simulink library "tenneco_lib"  (R2016b)
settings: Solver=ode45  StartTime=0.0  StopTime=10.0  RelTol=1e-3
undefined symbols (not defined in the file): Com_cntAMBInitTO_c, Com_cntAMBStopTO_c, Com_cntEC1InitTO_c, Com_cntEC1StopTO_c, Com_swAMBRx_c, Com_swEC1Rx_c, Com_swUseSPN108_c, Com_swUseSPN543_c, const, Env_pAmbPDflt_c, Env_pAmbPKOff_c, Env_pAmbPOvrd_c, Env_swAmbPOvrd_c, MSG_INIT_TIMEOUT, MSG_NOT_RECEIVED, MSG_RECEIVED_NOW, MSG_STOP_TIMEOUT
libraries: simulink x19, tenneco_lib x2
(part 3 of 5)

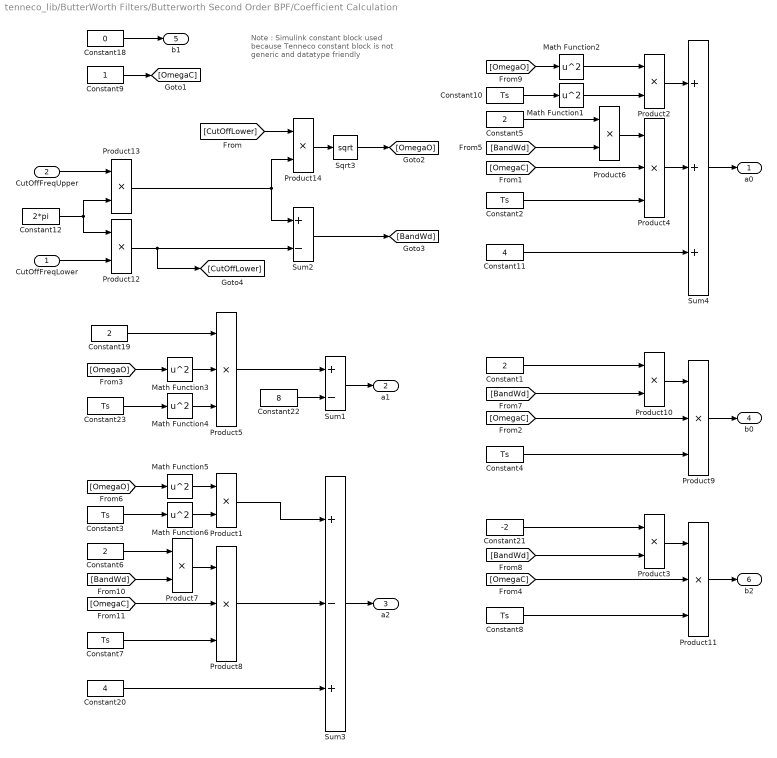
== system tenneco_lib/ButterWorth Filters/Butterworth Second Order BPF/Coefficient Calculation ==
  note: Note : Simulink constant block used because Tenneco constant block is not generic and datatype friendly
  CutOffFreqLower : Inport  mask(Standard Inport){Port=1}
      mask prompts: Port "Simulink:blkprm_prompts:InOutportPortNum"
      mask help: Provide an input port for subsystems.
      mask TypeOptions Port: Port
  CutOffFreqUpper : Inport  Port=2  mask(Standard Inport){Port=2}
      mask prompts: Port "Simulink:blkprm_prompts:InOutportPortNum"
      mask help: Provide an input port for subsystems.
      mask TypeOptions Port: Port
  Constant{1,5..6,19} (4 alike) : Constant  Value=2  OutDataTypeStr=Inherit: Inherit via back propagation
  Constant{2..4,7..8,10,23} (7 alike) : Constant  Value=Ts  OutDataTypeStr=Inherit: Inherit via back propagation
  Constant11 : Constant  Value=4  OutDataTypeStr=Inherit: Inherit via back propagation
  Constant12 : Constant  Value=2*pi  OutDataTypeStr=Inherit: Inherit via back propagation
  Constant18 : Constant  Value=0  OutDataTypeStr=Inherit: Inherit via back propagation
  Constant20 : Constant  Value=4  OutDataTypeStr=Inherit: Inherit via back propagation
  Constant21 : Constant  Value=-2  OutDataTypeStr=Inherit: Inherit via back propagation
  Constant22 : Constant  Value=8  OutDataTypeStr=Inherit: Inherit via back propagation
  Constant9 : Constant  OutDataTypeStr=Inherit: Inherit via back propagation
  Math Function1 : Math  Operator=square  SaturateOnIntegerOverflow=on  mask(Math){Operator=square}
      mask prompts: Operator "SimulinkBlocks:dialog:BmathfcnOperator"
      mask help: Mathematical functions including logarithmic, exponential, power, and modulus functions. When the function has more than one argument, the first argument corresponds to the top (or left) input port.
      mask TypeOptions Operator: Operator
  Math Function2 : Math  Operator=square  SaturateOnIntegerOverflow=on  mask(Math){Operator=square}
      mask prompts: Operator "SimulinkBlocks:dialog:BmathfcnOperator"
      mask help: Mathematical functions including logarithmic, exponential, power, and modulus functions. When the function has more than one argument, the first argument corresponds to the top (or left) input port.
      mask TypeOptions Operator: Operator
  Math Function3 : Math  Operator=square  SaturateOnIntegerOverflow=on  mask(Math){Operator=square}
      mask prompts: Operator "SimulinkBlocks:dialog:BmathfcnOperator"
      mask help: Mathematical functions including logarithmic, exponential, power, and modulus functions. When the function has more than one argument, the first argument corresponds to the top (or left) input port.
      mask TypeOptions Operator: Operator
  Math Function4 : Math  Operator=square  SaturateOnIntegerOverflow=on  mask(Math){Operator=square}
      mask prompts: Operator "SimulinkBlocks:dialog:BmathfcnOperator"
      mask help: Mathematical functions including logarithmic, exponential, power, and modulus functions. When the function has more than one argument, the first argument corresponds to the top (or left) input port.
      mask TypeOptions Operator: Operator
  Math Function5 : Math  Operator=square  SaturateOnIntegerOverflow=on  mask(Math){Operator=square}
      mask prompts: Operator "SimulinkBlocks:dialog:BmathfcnOperator"
      mask help: Mathematical functions including logarithmic, exponential, power, and modulus functions. When the function has more than one argument, the first argument corresponds to the top (or left) input port.
      mask TypeOptions Operator: Operator
  Math Function6 : Math  Operator=square  SaturateOnIntegerOverflow=on  mask(Math){Operator=square}
      mask prompts: Operator "SimulinkBlocks:dialog:BmathfcnOperator"
      mask help: Mathematical functions including logarithmic, exponential, power, and modulus functions. When the function has more than one argument, the first argument corresponds to the top (or left) input port.
      mask TypeOptions Operator: Operator
  Product1 : Product  Inputs=**  InputSameDT=on  mask(Product){Inputs=**}
      mask prompts: Inputs "List of signs:"
      mask help:
      | Multiply or divide inputs.  Specify one of the following:
      |  a) * or / for each input port. For example, **/* performs the operation 'u1*u2/u3*u4'.
      |  b) scalar specifies the number of input ports to be multiplied.
      mask TypeOptions Inputs: Inputs
  Product10 : Product  Inputs=**  InputSameDT=on  mask(Product){Inputs=**}
      mask prompts: Inputs "List of signs:"
      mask help:
      | Multiply or divide inputs.  Specify one of the following:
      |  a) * or / for each input port. For example, **/* performs the operation 'u1*u2/u3*u4'.
      |  b) scalar specifies the number of input ports to be multiplied.
      mask TypeOptions Inputs: Inputs
  Product11 : Product  Inputs=***  InputSameDT=on  mask(Product){Inputs=***}
      mask prompts: Inputs "List of signs:"
      mask help:
      | Multiply or divide inputs.  Specify one of the following:
      |  a) * or / for each input port. For example, **/* performs the operation 'u1*u2/u3*u4'.
      |  b) scalar specifies the number of input ports to be multiplied.
      mask TypeOptions Inputs: Inputs
  Product12 : Product  Inputs=**  InputSameDT=on  mask(Product){Inputs=**}
      mask prompts: Inputs "List of signs:"
      mask help:
      | Multiply or divide inputs.  Specify one of the following:
      |  a) * or / for each input port. For example, **/* performs the operation 'u1*u2/u3*u4'.
      |  b) scalar specifies the number of input ports to be multiplied.
      mask TypeOptions Inputs: Inputs
  Product13 : Product  Inputs=**  InputSameDT=on  mask(Product){Inputs=**}
      mask prompts: Inputs "List of signs:"
      mask help:
      | Multiply or divide inputs.  Specify one of the following:
      |  a) * or / for each input port. For example, **/* performs the operation 'u1*u2/u3*u4'.
      |  b) scalar specifies the number of input ports to be multiplied.
      mask TypeOptions Inputs: Inputs
  Product14 : Product  Inputs=**  InputSameDT=on  mask(Product){Inputs=**}
      mask prompts: Inputs "List of signs:"
      mask help:
      | Multiply or divide inputs.  Specify one of the following:
      |  a) * or / for each input port. For example, **/* performs the operation 'u1*u2/u3*u4'.
      |  b) scalar specifies the number of input ports to be multiplied.
      mask TypeOptions Inputs: Inputs
  Product2 : Product  Inputs=**  InputSameDT=on  mask(Product){Inputs=**}
      mask prompts: Inputs "List of signs:"
      mask help:
      | Multiply or divide inputs.  Specify one of the following:
      |  a) * or / for each input port. For example, **/* performs the operation 'u1*u2/u3*u4'.
      |  b) scalar specifies the number of input ports to be multiplied.
      mask TypeOptions Inputs: Inputs
  Product3 : Product  Inputs=**  InputSameDT=on  mask(Product){Inputs=**}
      mask prompts: Inputs "List of signs:"
      mask help:
      | Multiply or divide inputs.  Specify one of the following:
      |  a) * or / for each input port. For example, **/* performs the operation 'u1*u2/u3*u4'.
      |  b) scalar specifies the number of input ports to be multiplied.
      mask TypeOptions Inputs: Inputs
  Product4 : Product  Inputs=***  InputSameDT=on  mask(Product){Inputs=***}
      mask prompts: Inputs "List of signs:"
      mask help:
      | Multiply or divide inputs.  Specify one of the following:
      |  a) * or / for each input port. For example, **/* performs the operation 'u1*u2/u3*u4'.
      |  b) scalar specifies the number of input ports to be multiplied.
      mask TypeOptions Inputs: Inputs
  Product5 : Product  Inputs=***  InputSameDT=on  mask(Product){Inputs=***}
      mask prompts: Inputs "List of signs:"
      mask help:
      | Multiply or divide inputs.  Specify one of the following:
      |  a) * or / for each input port. For example, **/* performs the operation 'u1*u2/u3*u4'.
      |  b) scalar specifies the number of input ports to be multiplied.
      mask TypeOptions Inputs: Inputs
  Product6 : Product  Inputs=**  InputSameDT=on  mask(Product){Inputs=**}
      mask prompts: Inputs "List of signs:"
      mask help:
      | Multiply or divide inputs.  Specify one of the following:
      |  a) * or / for each input port. For example, **/* performs the operation 'u1*u2/u3*u4'.
      |  b) scalar specifies the number of input ports to be multiplied.
      mask TypeOptions Inputs: Inputs
  Product7 : Product  Inputs=**  InputSameDT=on  mask(Product){Inputs=**}
      mask prompts: Inputs "List of signs:"
      mask help:
      | Multiply or divide inputs.  Specify one of the following:
      |  a) * or / for each input port. For example, **/* performs the operation 'u1*u2/u3*u4'.
      |  b) scalar specifies the number of input ports to be multiplied.
      mask TypeOptions Inputs: Inputs
  Product8 : Product  Inputs=***  InputSameDT=on  mask(Product){Inputs=***}
      mask prompts: Inputs "List of signs:"
      mask help:
      | Multiply or divide inputs.  Specify one of the following:
      |  a) * or / for each input port. For example, **/* performs the operation 'u1*u2/u3*u4'.
      |  b) scalar specifies the number of input ports to be multiplied.
      mask TypeOptions Inputs: Inputs
  Product9 : Product  Inputs=***  InputSameDT=on  mask(Product){Inputs=***}
      mask prompts: Inputs "List of signs:"
      mask help:
      | Multiply or divide inputs.  Specify one of the following:
      |  a) * or / for each input port. For example, **/* performs the operation 'u1*u2/u3*u4'.
      |  b) scalar specifies the number of input ports to be multiplied.
      mask TypeOptions Inputs: Inputs
  Sqrt3 : Sqrt  SaturateOnIntegerOverflow=on  mask(Sqrt){Operator=sqrt}
      mask prompts: Operator "SimulinkBlocks:SqrtFcn:BmathfcnOperator"
      mask help: Square root functions including square root, signed square root, and reciprocal square root functions.
      mask TypeOptions Operator: Operator
  Sum1 : Sum  Inputs=+-  InputSameDT=on  mask(Sum){Inputs=+-}
      mask prompts: Inputs "Simulink:blkprm_prompts:SumListofSigns"
      mask help:
      | Add or subtract inputs.  Specify one of the following:
      | a) character vector containing + or - for each input port, | for spacer between ports (e.g. ++|-|++)
      | b) scalar, >= 1, specifies the number of input ports to be summed.
      | When there is only one input port, add or subtract elements over all dimensions or one specified dimension
      mask TypeOptions Inputs: Inputs
  Sum2 : Sum  Inputs=+-  InputSameDT=on  mask(Sum){Inputs=+-}
      mask prompts: Inputs "Simulink:blkprm_prompts:SumListofSigns"
      mask help:
      | Add or subtract inputs.  Specify one of the following:
      | a) character vector containing + or - for each input port, | for spacer between ports (e.g. ++|-|++)
      | b) scalar, >= 1, specifies the number of input ports to be summed.
      | When there is only one input port, add or subtract elements over all dimensions or one specified dimension
      mask TypeOptions Inputs: Inputs
  Sum3 : Sum  Inputs=+-+  InputSameDT=on  mask(Sum){Inputs=+-+}
      mask prompts: Inputs "Simulink:blkprm_prompts:SumListofSigns"
      mask help:
      | Add or subtract inputs.  Specify one of the following:
      | a) character vector containing + or - for each input port, | for spacer between ports (e.g. ++|-|++)
      | b) scalar, >= 1, specifies the number of input ports to be summed.
      | When there is only one input port, add or subtract elements over all dimensions or one specified dimension
      mask TypeOptions Inputs: Inputs
  Sum4 : Sum  Inputs=+++  InputSameDT=on  mask(Sum){Inputs=+++}
      mask prompts: Inputs "Simulink:blkprm_prompts:SumListofSigns"
      mask help:
      | Add or subtract inputs.  Specify one of the following:
      | a) character vector containing + or - for each input port, | for spacer between ports (e.g. ++|-|++)
      | b) scalar, >= 1, specifies the number of input ports to be summed.
      | When there is only one input port, add or subtract elements over all dimensions or one specified dimension
      mask TypeOptions Inputs: Inputs
  a0 : Outport  mask(Standard Outport){Port=1}
      mask prompts: Port "Simulink:blkprm_prompts:InOutportPortNum"
      mask help: Provide an output port for subsystems.
      mask TypeOptions Port: Port
  a1 : Outport  Port=2  mask(Standard Outport){Port=2}
      mask prompts: Port "Simulink:blkprm_prompts:InOutportPortNum"
      mask help: Provide an output port for subsystems.
      mask TypeOptions Port: Port
  a2 : Outport  Port=3  mask(Standard Outport){Port=3}
      mask prompts: Port "Simulink:blkprm_prompts:InOutportPortNum"
      mask help: Provide an output port for subsystems.
      mask TypeOptions Port: Port
  b0 : Outport  Port=4  mask(Standard Outport){Port=4}
      mask prompts: Port "Simulink:blkprm_prompts:InOutportPortNum"
      mask help: Provide an output port for subsystems.
      mask TypeOptions Port: Port
  b1 : Outport  Port=5  mask(Standard Outport){Port=5}
      mask prompts: Port "Simulink:blkprm_prompts:InOutportPortNum"
      mask help: Provide an output port for subsystems.
      mask TypeOptions Port: Port
  b2 : Outport  Port=6  mask(Standard Outport){Port=6}
      mask prompts: Port "Simulink:blkprm_prompts:InOutportPortNum"
      mask help: Provide an output port for subsystems.
      mask TypeOptions Port: Port
  wires:
  Constant18/1 -> b1/1
  Sum1/1 -> a1/1
  Constant9/1 -> [OmegaC]
  [OmegaO] -> Math Function2/1
  Product2/1 -> Sum4/1
  Math Function2/1 -> Product2/1
  Math Function1/1 -> Product2/2
  Constant10/1 -> Math Function1/1
  Constant11/1 -> Sum4/3
  Product4/1 -> Sum4/2
  [OmegaC] -> Product4/2
  Constant2/1 -> Product4/3
  Product6/1 -> Product4/1
  Constant5/1 -> Product6/1
  [BandWd] -> Product6/2
  Sum4/1 -> a0/1
  Constant22/1 -> Sum1/2
  [OmegaO] -> Math Function3/1
  Product5/1 -> Sum1/1
  Constant23/1 -> Math Function4/1
  Math Function3/1 -> Product5/2
  Math Function4/1 -> Product5/3
  Constant19/1 -> Product5/1
  [OmegaO] -> Math Function5/1
  Product1/1 -> Sum3/1
  Math Function5/1 -> Product1/1
  Math Function6/1 -> Product1/2
  Constant3/1 -> Math Function6/1
  Constant20/1 -> Sum3/3
  Product8/1 -> Sum3/2
  [OmegaC] -> Product8/2
  Constant7/1 -> Product8/3
  Product7/1 -> Product8/1
  Constant6/1 -> Product7/1
  [BandWd] -> Product7/2
  Sum3/1 -> a2/1
  Product9/1 -> b0/1
  [OmegaC] -> Product9/2
  Constant4/1 -> Product9/3
  Product10/1 -> Product9/1
  [BandWd] -> Product10/2
  Constant1/1 -> Product10/1
  Product11/1 -> b2/1
  [OmegaC] -> Product11/2
  Constant8/1 -> Product11/3
  Product3/1 -> Product11/1
  [BandWd] -> Product3/2
  Constant21/1 -> Product3/1
  Sqrt3/1 -> [OmegaO]
  Product14/1 -> Sqrt3/1
  [CutOffLower] -> Product14/1
  Sum2/1 -> [BandWd]
  Product12/1 -> Sum2/2, [CutOffLower]
  Product13/1 -> Sum2/1, Product14/2
  CutOffFreqLower/1 -> Product12/2
  CutOffFreqUpper/1 -> Product13/1
  Constant12/1 -> Product13/2, Product12/1

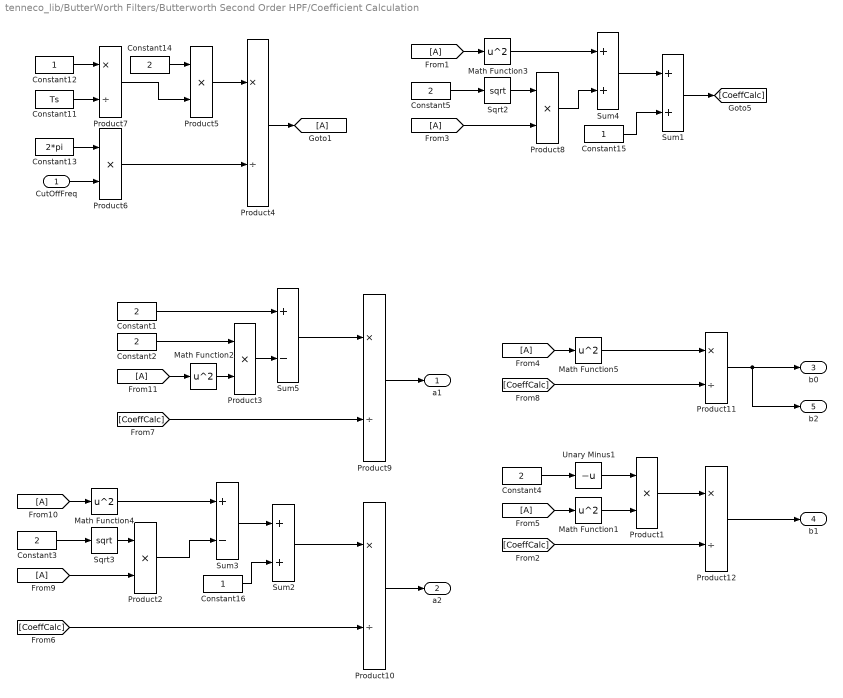
== system tenneco_lib/ButterWorth Filters/Butterworth Second Order HPF/Coefficient Calculation ==
  CutOffFreq : Inport  mask(Standard Inport){Port=1}
      mask prompts: Port "Simulink:blkprm_prompts:InOutportPortNum"
      mask help: Provide an input port for subsystems.
      mask TypeOptions Port: Port
  Constant{1..5,14} (6 alike) : Constant  Value=2  OutDataTypeStr=Inherit: Inherit via back propagation
  Constant11 : Constant  Value=Ts  OutDataTypeStr=Inherit: Inherit via back propagation
  Constant12 : Constant  OutDataTypeStr=Inherit: Inherit via back propagation
  Constant13 : Constant  Value=2*pi  OutDataTypeStr=Inherit: Inherit via back propagation
  Constant15 : Constant  OutDataTypeStr=Inherit: Inherit via back propagation
  Constant16 : Constant  OutDataTypeStr=Inherit: Inherit via back propagation
  Math Function1 : Math  Operator=square  SaturateOnIntegerOverflow=on  mask(Math){Operator=square}
      mask prompts: Operator "SimulinkBlocks:dialog:BmathfcnOperator"
      mask help: Mathematical functions including logarithmic, exponential, power, and modulus functions. When the function has more than one argument, the first argument corresponds to the top (or left) input port.
      mask TypeOptions Operator: Operator
  Math Function2 : Math  Operator=square  SaturateOnIntegerOverflow=on  mask(Math){Operator=square}
      mask prompts: Operator "SimulinkBlocks:dialog:BmathfcnOperator"
      mask help: Mathematical functions including logarithmic, exponential, power, and modulus functions. When the function has more than one argument, the first argument corresponds to the top (or left) input port.
      mask TypeOptions Operator: Operator
  Math Function3 : Math  Operator=square  SaturateOnIntegerOverflow=on  mask(Math){Operator=square}
      mask prompts: Operator "SimulinkBlocks:dialog:BmathfcnOperator"
      mask help: Mathematical functions including logarithmic, exponential, power, and modulus functions. When the function has more than one argument, the first argument corresponds to the top (or left) input port.
      mask TypeOptions Operator: Operator
  Math Function4 : Math  Operator=square  SaturateOnIntegerOverflow=on  mask(Math){Operator=square}
      mask prompts: Operator "SimulinkBlocks:dialog:BmathfcnOperator"
      mask help: Mathematical functions including logarithmic, exponential, power, and modulus functions. When the function has more than one argument, the first argument corresponds to the top (or left) input port.
      mask TypeOptions Operator: Operator
  Math Function5 : Math  Operator=square  SaturateOnIntegerOverflow=on  mask(Math){Operator=square}
      mask prompts: Operator "SimulinkBlocks:dialog:BmathfcnOperator"
      mask help: Mathematical functions including logarithmic, exponential, power, and modulus functions. When the function has more than one argument, the first argument corresponds to the top (or left) input port.
      mask TypeOptions Operator: Operator
  Product1 : Product  Inputs=**  InputSameDT=on  mask(Product){Inputs=**}
      mask prompts: Inputs "List of signs:"
      mask help:
      | Multiply or divide inputs.  Specify one of the following:
      |  a) * or / for each input port. For example, **/* performs the operation 'u1*u2/u3*u4'.
      |  b) scalar specifies the number of input ports to be multiplied.
      mask TypeOptions Inputs: Inputs
  Product10 : Product  Inputs=*/  InputSameDT=on  mask(Product){Inputs=*/}
      mask prompts: Inputs "List of signs:"
      mask help:
      | Multiply or divide inputs.  Specify one of the following:
      |  a) * or / for each input port. For example, **/* performs the operation 'u1*u2/u3*u4'.
      |  b) scalar specifies the number of input ports to be multiplied.
      mask TypeOptions Inputs: Inputs
  Product11 : Product  Inputs=*/  InputSameDT=on  mask(Product){Inputs=*/}
      mask prompts: Inputs "List of signs:"
      mask help:
      | Multiply or divide inputs.  Specify one of the following:
      |  a) * or / for each input port. For example, **/* performs the operation 'u1*u2/u3*u4'.
      |  b) scalar specifies the number of input ports to be multiplied.
      mask TypeOptions Inputs: Inputs
  Product12 : Product  Inputs=*/  InputSameDT=on  mask(Product){Inputs=*/}
      mask prompts: Inputs "List of signs:"
      mask help:
      | Multiply or divide inputs.  Specify one of the following:
      |  a) * or / for each input port. For example, **/* performs the operation 'u1*u2/u3*u4'.
      |  b) scalar specifies the number of input ports to be multiplied.
      mask TypeOptions Inputs: Inputs
  Product2 : Product  Inputs=**  InputSameDT=on  mask(Product){Inputs=**}
      mask prompts: Inputs "List of signs:"
      mask help:
      | Multiply or divide inputs.  Specify one of the following:
      |  a) * or / for each input port. For example, **/* performs the operation 'u1*u2/u3*u4'.
      |  b) scalar specifies the number of input ports to be multiplied.
      mask TypeOptions Inputs: Inputs
  Product3 : Product  Inputs=**  InputSameDT=on  mask(Product){Inputs=**}
      mask prompts: Inputs "List of signs:"
      mask help:
      | Multiply or divide inputs.  Specify one of the following:
      |  a) * or / for each input port. For example, **/* performs the operation 'u1*u2/u3*u4'.
      |  b) scalar specifies the number of input ports to be multiplied.
      mask TypeOptions Inputs: Inputs
  Product4 : Product  Inputs=*/  InputSameDT=on  mask(Product){Inputs=*/}
      mask prompts: Inputs "List of signs:"
      mask help:
      | Multiply or divide inputs.  Specify one of the following:
      |  a) * or / for each input port. For example, **/* performs the operation 'u1*u2/u3*u4'.
      |  b) scalar specifies the number of input ports to be multiplied.
      mask TypeOptions Inputs: Inputs
  Product5 : Product  Inputs=**  InputSameDT=on  mask(Product){Inputs=**}
      mask prompts: Inputs "List of signs:"
      mask help:
      | Multiply or divide inputs.  Specify one of the following:
      |  a) * or / for each input port. For example, **/* performs the operation 'u1*u2/u3*u4'.
      |  b) scalar specifies the number of input ports to be multiplied.
      mask TypeOptions Inputs: Inputs
  Product6 : Product  Inputs=**  InputSameDT=on  mask(Product){Inputs=**}
      mask prompts: Inputs "List of signs:"
      mask help:
      | Multiply or divide inputs.  Specify one of the following:
      |  a) * or / for each input port. For example, **/* performs the operation 'u1*u2/u3*u4'.
      |  b) scalar specifies the number of input ports to be multiplied.
      mask TypeOptions Inputs: Inputs
  Product7 : Product  Inputs=*/  InputSameDT=on  mask(Product){Inputs=*/}
      mask prompts: Inputs "List of signs:"
      mask help:
      | Multiply or divide inputs.  Specify one of the following:
      |  a) * or / for each input port. For example, **/* performs the operation 'u1*u2/u3*u4'.
      |  b) scalar specifies the number of input ports to be multiplied.
      mask TypeOptions Inputs: Inputs
  Product8 : Product  Inputs=**  InputSameDT=on  mask(Product){Inputs=**}
      mask prompts: Inputs "List of signs:"
      mask help:
      | Multiply or divide inputs.  Specify one of the following:
      |  a) * or / for each input port. For example, **/* performs the operation 'u1*u2/u3*u4'.
      |  b) scalar specifies the number of input ports to be multiplied.
      mask TypeOptions Inputs: Inputs
  Product9 : Product  Inputs=*/  InputSameDT=on  mask(Product){Inputs=*/}
      mask prompts: Inputs "List of signs:"
      mask help:
      | Multiply or divide inputs.  Specify one of the following:
      |  a) * or / for each input port. For example, **/* performs the operation 'u1*u2/u3*u4'.
      |  b) scalar specifies the number of input ports to be multiplied.
      mask TypeOptions Inputs: Inputs
  Sqrt2 : Sqrt  SaturateOnIntegerOverflow=on  mask(Sqrt){Operator=sqrt}
      mask prompts: Operator "SimulinkBlocks:SqrtFcn:BmathfcnOperator"
      mask help: Square root functions including square root, signed square root, and reciprocal square root functions.
      mask TypeOptions Operator: Operator
  Sqrt3 : Sqrt  SaturateOnIntegerOverflow=on  mask(Sqrt){Operator=sqrt}
      mask prompts: Operator "SimulinkBlocks:SqrtFcn:BmathfcnOperator"
      mask help: Square root functions including square root, signed square root, and reciprocal square root functions.
      mask TypeOptions Operator: Operator
  Sum1 : Sum  InputSameDT=on  mask(Sum){Inputs=++}
      mask prompts: Inputs "Simulink:blkprm_prompts:SumListofSigns"
      mask help:
      | Add or subtract inputs.  Specify one of the following:
      | a) character vector containing + or - for each input port, | for spacer between ports (e.g. ++|-|++)
      | b) scalar, >= 1, specifies the number of input ports to be summed.
      | When there is only one input port, add or subtract elements over all dimensions or one specified dimension
      mask TypeOptions Inputs: Inputs
  Sum2 : Sum  InputSameDT=on  mask(Sum){Inputs=++}
      mask prompts: Inputs "Simulink:blkprm_prompts:SumListofSigns"
      mask help:
      | Add or subtract inputs.  Specify one of the following:
      | a) character vector containing + or - for each input port, | for spacer between ports (e.g. ++|-|++)
      | b) scalar, >= 1, specifies the number of input ports to be summed.
      | When there is only one input port, add or subtract elements over all dimensions or one specified dimension
      mask TypeOptions Inputs: Inputs
  Sum3 : Sum  Inputs=+-  InputSameDT=on  mask(Sum){Inputs=+-}
      mask prompts: Inputs "Simulink:blkprm_prompts:SumListofSigns"
      mask help:
      | Add or subtract inputs.  Specify one of the following:
      | a) character vector containing + or - for each input port, | for spacer between ports (e.g. ++|-|++)
      | b) scalar, >= 1, specifies the number of input ports to be summed.
      | When there is only one input port, add or subtract elements over all dimensions or one specified dimension
      mask TypeOptions Inputs: Inputs
  Sum4 : Sum  InputSameDT=on  mask(Sum){Inputs=++}
      mask prompts: Inputs "Simulink:blkprm_prompts:SumListofSigns"
      mask help:
      | Add or subtract inputs.  Specify one of the following:
      | a) character vector containing + or - for each input port, | for spacer between ports (e.g. ++|-|++)
      | b) scalar, >= 1, specifies the number of input ports to be summed.
      | When there is only one input port, add or subtract elements over all dimensions or one specified dimension
      mask TypeOptions Inputs: Inputs
  Sum5 : Sum  Inputs=+-  InputSameDT=on  mask(Sum){Inputs=+-}
      mask prompts: Inputs "Simulink:blkprm_prompts:SumListofSigns"
      mask help:
      | Add or subtract inputs.  Specify one of the following:
      | a) character vector containing + or - for each input port, | for spacer between ports (e.g. ++|-|++)
      | b) scalar, >= 1, specifies the number of input ports to be summed.
      | When there is only one input port, add or subtract elements over all dimensions or one specified dimension
      mask TypeOptions Inputs: Inputs
  Unary Minus1 : UnaryMinus
  a1 : Outport  mask(Standard Outport){Port=1}
      mask prompts: Port "Simulink:blkprm_prompts:InOutportPortNum"
      mask help: Provide an output port for subsystems.
      mask TypeOptions Port: Port
  a2 : Outport  Port=2  mask(Standard Outport){Port=2}
      mask prompts: Port "Simulink:blkprm_prompts:InOutportPortNum"
      mask help: Provide an output port for subsystems.
      mask TypeOptions Port: Port
  b0 : Outport  Port=3  mask(Standard Outport){Port=3}
      mask prompts: Port "Simulink:blkprm_prompts:InOutportPortNum"
      mask help: Provide an output port for subsystems.
      mask TypeOptions Port: Port
  b1 : Outport  Port=4  mask(Standard Outport){Port=4}
      mask prompts: Port "Simulink:blkprm_prompts:InOutportPortNum"
      mask help: Provide an output port for subsystems.
      mask TypeOptions Port: Port
  b2 : Outport  Port=5  mask(Standard Outport){Port=5}
      mask prompts: Port "Simulink:blkprm_prompts:InOutportPortNum"
      mask help: Provide an output port for subsystems.
      mask TypeOptions Port: Port
  wires:
  Constant14/1 -> Product5/1
  Product7/1 -> Product5/2
  Product5/1 -> Product4/1
  Product4/1 -> [A]
  Product6/1 -> Product4/2
  Constant13/1 -> Product6/1
  Constant12/1 -> Product7/1
  CutOffFreq/1 -> Product6/2
  Constant11/1 -> Product7/2
  Unary Minus1/1 -> Product1/1
  Constant4/1 -> Unary Minus1/1
  Math Function1/1 -> Product1/2
  [A] -> Math Function1/1
  [A] -> Math Function5/1
  Product1/1 -> Product12/1
  [CoeffCalc] -> Product12/2
  Product12/1 -> b1/1
  [CoeffCalc] -> Product11/2
  [CoeffCalc] -> Product10/2
  [CoeffCalc] -> Product9/2
  Sum1/1 -> [CoeffCalc]
  Product10/1 -> a2/1
  Sum2/1 -> Product10/1
  Constant16/1 -> Sum2/2
  Sum3/1 -> Sum2/1
  Math Function4/1 -> Sum3/1
  Product2/1 -> Sum3/2
  [A] -> Product2/2
  Sqrt3/1 -> Product2/1
  Constant3/1 -> Sqrt3/1
  [A] -> Math Function4/1
  Product9/1 -> a1/1
  Constant15/1 -> Sum1/2
  Sum4/1 -> Sum1/1
  Math Function3/1 -> Sum4/1
  Product8/1 -> Sum4/2
  [A] -> Product8/2
  Sqrt2/1 -> Product8/1
  Constant5/1 -> Sqrt2/1
  [A] -> Math Function3/1
  Sum5/1 -> Product9/1
  Product3/1 -> Sum5/2
  Constant2/1 -> Product3/1
  Math Function2/1 -> Product3/2
  [A] -> Math Function2/1
  Constant1/1 -> Sum5/1
  Math Function5/1 -> Product11/1
  Product11/1 -> b2/1, b0/1

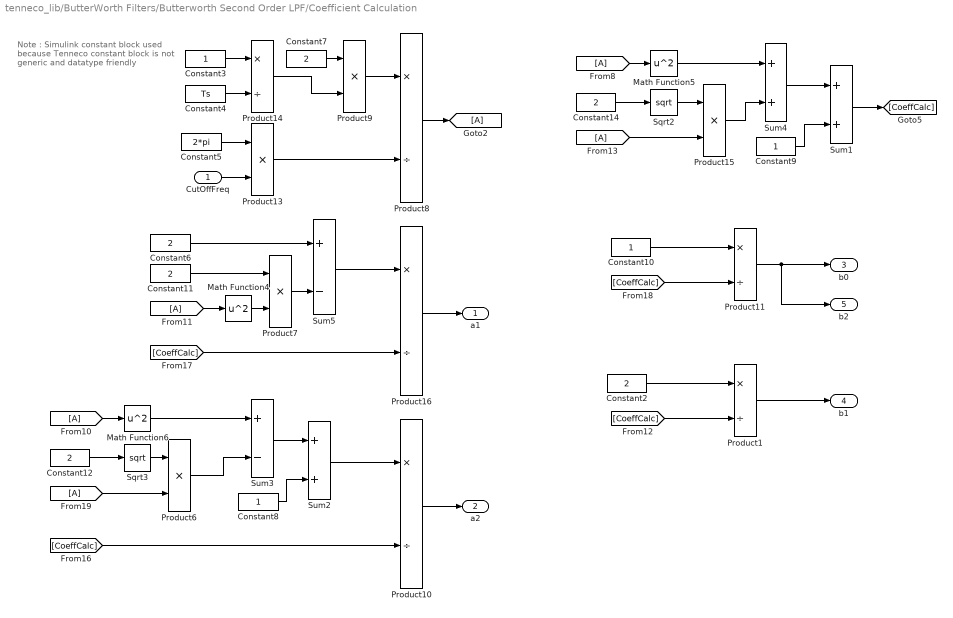
== system tenneco_lib/ButterWorth Filters/Butterworth Second Order LPF/Coefficient Calculation ==
  note: Note : Simulink constant block used because Tenneco constant block is not generic and datatype friendly
  CutOffFreq : Inport  mask(Standard Inport){Port=1}
      mask prompts: Port "Simulink:blkprm_prompts:InOutportPortNum"
      mask help: Provide an input port for subsystems.
      mask TypeOptions Port: Port
  Constant{3,8..10} (4 alike) : Constant  OutDataTypeStr=Inherit: Inherit via back propagation
  Constant{2,6..7,11..12,14} (6 alike) : Constant  Value=2  OutDataTypeStr=Inherit: Inherit via back propagation
  Constant4 : Constant  Value=Ts  OutDataTypeStr=Inherit: Inherit via back propagation
  Constant5 : Constant  Value=2*pi  OutDataTypeStr=Inherit: Inherit via back propagation
  Math Function4 : Math  Operator=square  SaturateOnIntegerOverflow=on  mask(Math){Operator=square}
      mask prompts: Operator "SimulinkBlocks:dialog:BmathfcnOperator"
      mask help: Mathematical functions including logarithmic, exponential, power, and modulus functions. When the function has more than one argument, the first argument corresponds to the top (or left) input port.
      mask TypeOptions Operator: Operator
  Math Function5 : Math  Operator=square  SaturateOnIntegerOverflow=on  mask(Math){Operator=square}
      mask prompts: Operator "SimulinkBlocks:dialog:BmathfcnOperator"
      mask help: Mathematical functions including logarithmic, exponential, power, and modulus functions. When the function has more than one argument, the first argument corresponds to the top (or left) input port.
      mask TypeOptions Operator: Operator
  Math Function6 : Math  Operator=square  SaturateOnIntegerOverflow=on  mask(Math){Operator=square}
      mask prompts: Operator "SimulinkBlocks:dialog:BmathfcnOperator"
      mask help: Mathematical functions including logarithmic, exponential, power, and modulus functions. When the function has more than one argument, the first argument corresponds to the top (or left) input port.
      mask TypeOptions Operator: Operator
  Product1 : Product  Inputs=*/  InputSameDT=on  mask(Product){Inputs=*/}
      mask prompts: Inputs "List of signs:"
      mask help:
      | Multiply or divide inputs.  Specify one of the following:
      |  a) * or / for each input port. For example, **/* performs the operation 'u1*u2/u3*u4'.
      |  b) scalar specifies the number of input ports to be multiplied.
      mask TypeOptions Inputs: Inputs
  Product10 : Product  Inputs=*/  InputSameDT=on  mask(Product){Inputs=*/}
      mask prompts: Inputs "List of signs:"
      mask help:
      | Multiply or divide inputs.  Specify one of the following:
      |  a) * or / for each input port. For example, **/* performs the operation 'u1*u2/u3*u4'.
      |  b) scalar specifies the number of input ports to be multiplied.
      mask TypeOptions Inputs: Inputs
  Product11 : Product  Inputs=*/  InputSameDT=on  mask(Product){Inputs=*/}
      mask prompts: Inputs "List of signs:"
      mask help:
      | Multiply or divide inputs.  Specify one of the following:
      |  a) * or / for each input port. For example, **/* performs the operation 'u1*u2/u3*u4'.
      |  b) scalar specifies the number of input ports to be multiplied.
      mask TypeOptions Inputs: Inputs
  Product13 : Product  Inputs=**  InputSameDT=on  mask(Product){Inputs=**}
      mask prompts: Inputs "List of signs:"
      mask help:
      | Multiply or divide inputs.  Specify one of the following:
      |  a) * or / for each input port. For example, **/* performs the operation 'u1*u2/u3*u4'.
      |  b) scalar specifies the number of input ports to be multiplied.
      mask TypeOptions Inputs: Inputs
  Product14 : Product  Inputs=*/  InputSameDT=on  mask(Product){Inputs=*/}
      mask prompts: Inputs "List of signs:"
      mask help:
      | Multiply or divide inputs.  Specify one of the following:
      |  a) * or / for each input port. For example, **/* performs the operation 'u1*u2/u3*u4'.
      |  b) scalar specifies the number of input ports to be multiplied.
      mask TypeOptions Inputs: Inputs
  Product15 : Product  Inputs=**  InputSameDT=on  mask(Product){Inputs=**}
      mask prompts: Inputs "List of signs:"
      mask help:
      | Multiply or divide inputs.  Specify one of the following:
      |  a) * or / for each input port. For example, **/* performs the operation 'u1*u2/u3*u4'.
      |  b) scalar specifies the number of input ports to be multiplied.
      mask TypeOptions Inputs: Inputs
  Product16 : Product  Inputs=*/  InputSameDT=on  mask(Product){Inputs=*/}
      mask prompts: Inputs "List of signs:"
      mask help:
      | Multiply or divide inputs.  Specify one of the following:
      |  a) * or / for each input port. For example, **/* performs the operation 'u1*u2/u3*u4'.
      |  b) scalar specifies the number of input ports to be multiplied.
      mask TypeOptions Inputs: Inputs
  Product6 : Product  Inputs=**  InputSameDT=on  mask(Product){Inputs=**}
      mask prompts: Inputs "List of signs:"
      mask help:
      | Multiply or divide inputs.  Specify one of the following:
      |  a) * or / for each input port. For example, **/* performs the operation 'u1*u2/u3*u4'.
      |  b) scalar specifies the number of input ports to be multiplied.
      mask TypeOptions Inputs: Inputs
  Product7 : Product  Inputs=**  InputSameDT=on  mask(Product){Inputs=**}
      mask prompts: Inputs "List of signs:"
      mask help:
      | Multiply or divide inputs.  Specify one of the following:
      |  a) * or / for each input port. For example, **/* performs the operation 'u1*u2/u3*u4'.
      |  b) scalar specifies the number of input ports to be multiplied.
      mask TypeOptions Inputs: Inputs
  Product8 : Product  Inputs=*/  InputSameDT=on  mask(Product){Inputs=*/}
      mask prompts: Inputs "List of signs:"
      mask help:
      | Multiply or divide inputs.  Specify one of the following:
      |  a) * or / for each input port. For example, **/* performs the operation 'u1*u2/u3*u4'.
      |  b) scalar specifies the number of input ports to be multiplied.
      mask TypeOptions Inputs: Inputs
  Product9 : Product  Inputs=**  InputSameDT=on  mask(Product){Inputs=**}
      mask prompts: Inputs "List of signs:"
      mask help:
      | Multiply or divide inputs.  Specify one of the following:
      |  a) * or / for each input port. For example, **/* performs the operation 'u1*u2/u3*u4'.
      |  b) scalar specifies the number of input ports to be multiplied.
      mask TypeOptions Inputs: Inputs
  Sqrt2 : Sqrt  SaturateOnIntegerOverflow=on  mask(Sqrt){Operator=sqrt}
      mask prompts: Operator "SimulinkBlocks:SqrtFcn:BmathfcnOperator"
      mask help: Square root functions including square root, signed square root, and reciprocal square root functions.
      mask TypeOptions Operator: Operator
  Sqrt3 : Sqrt  SaturateOnIntegerOverflow=on  mask(Sqrt){Operator=sqrt}
      mask prompts: Operator "SimulinkBlocks:SqrtFcn:BmathfcnOperator"
      mask help: Square root functions including square root, signed square root, and reciprocal square root functions.
      mask TypeOptions Operator: Operator
  Sum1 : Sum  InputSameDT=on  mask(Sum){Inputs=++}
      mask prompts: Inputs "Simulink:blkprm_prompts:SumListofSigns"
      mask help:
      | Add or subtract inputs.  Specify one of the following:
      | a) character vector containing + or - for each input port, | for spacer between ports (e.g. ++|-|++)
      | b) scalar, >= 1, specifies the number of input ports to be summed.
      | When there is only one input port, add or subtract elements over all dimensions or one specified dimension
      mask TypeOptions Inputs: Inputs
  Sum2 : Sum  InputSameDT=on  mask(Sum){Inputs=++}
      mask prompts: Inputs "Simulink:blkprm_prompts:SumListofSigns"
      mask help:
      | Add or subtract inputs.  Specify one of the following:
      | a) character vector containing + or - for each input port, | for spacer between ports (e.g. ++|-|++)
      | b) scalar, >= 1, specifies the number of input ports to be summed.
      | When there is only one input port, add or subtract elements over all dimensions or one specified dimension
      mask TypeOptions Inputs: Inputs
  Sum3 : Sum  Inputs=+-  InputSameDT=on  mask(Sum){Inputs=+-}
      mask prompts: Inputs "Simulink:blkprm_prompts:SumListofSigns"
      mask help:
      | Add or subtract inputs.  Specify one of the following:
      | a) character vector containing + or - for each input port, | for spacer between ports (e.g. ++|-|++)
      | b) scalar, >= 1, specifies the number of input ports to be summed.
      | When there is only one input port, add or subtract elements over all dimensions or one specified dimension
      mask TypeOptions Inputs: Inputs
  Sum4 : Sum  InputSameDT=on  mask(Sum){Inputs=++}
      mask prompts: Inputs "Simulink:blkprm_prompts:SumListofSigns"
      mask help:
      | Add or subtract inputs.  Specify one of the following:
      | a) character vector containing + or - for each input port, | for spacer between ports (e.g. ++|-|++)
      | b) scalar, >= 1, specifies the number of input ports to be summed.
      | When there is only one input port, add or subtract elements over all dimensions or one specified dimension
      mask TypeOptions Inputs: Inputs
  Sum5 : Sum  Inputs=+-  InputSameDT=on  mask(Sum){Inputs=+-}
      mask prompts: Inputs "Simulink:blkprm_prompts:SumListofSigns"
      mask help:
      | Add or subtract inputs.  Specify one of the following:
      | a) character vector containing + or - for each input port, | for spacer between ports (e.g. ++|-|++)
      | b) scalar, >= 1, specifies the number of input ports to be summed.
      | When there is only one input port, add or subtract elements over all dimensions or one specified dimension
      mask TypeOptions Inputs: Inputs
  a1 : Outport  mask(Standard Outport){Port=1}
      mask prompts: Port "Simulink:blkprm_prompts:InOutportPortNum"
      mask help: Provide an output port for subsystems.
      mask TypeOptions Port: Port
  a2 : Outport  Port=2  mask(Standard Outport){Port=2}
      mask prompts: Port "Simulink:blkprm_prompts:InOutportPortNum"
      mask help: Provide an output port for subsystems.
      mask TypeOptions Port: Port
  b0 : Outport  Port=3  mask(Standard Outport){Port=3}
      mask prompts: Port "Simulink:blkprm_prompts:InOutportPortNum"
      mask help: Provide an output port for subsystems.
      mask TypeOptions Port: Port
  b1 : Outport  Port=4  mask(Standard Outport){Port=4}
      mask prompts: Port "Simulink:blkprm_prompts:InOutportPortNum"
      mask help: Provide an output port for subsystems.
      mask TypeOptions Port: Port
  b2 : Outport  Port=5  mask(Standard Outport){Port=5}
      mask prompts: Port "Simulink:blkprm_prompts:InOutportPortNum"
      mask help: Provide an output port for subsystems.
      mask TypeOptions Port: Port
  wires:
  Constant7/1 -> Product9/1
  Product14/1 -> Product9/2
  Product9/1 -> Product8/1
  Product8/1 -> [A]
  Product13/1 -> Product8/2
  Constant5/1 -> Product13/1
  Constant3/1 -> Product14/1
  CutOffFreq/1 -> Product13/2
  Constant4/1 -> Product14/2
  [CoeffCalc] -> Product1/2
  Product1/1 -> b1/1
  [CoeffCalc] -> Product11/2
  [CoeffCalc] -> Product10/2
  [CoeffCalc] -> Product16/2
  Sum1/1 -> [CoeffCalc]
  Product10/1 -> a2/1
  Sum2/1 -> Product10/1
  Constant8/1 -> Sum2/2
  Sum3/1 -> Sum2/1
  Math Function6/1 -> Sum3/1
  Product6/1 -> Sum3/2
  [A] -> Product6/2
  Sqrt3/1 -> Product6/1
  Constant12/1 -> Sqrt3/1
  [A] -> Math Function6/1
  Product16/1 -> a1/1
  Constant9/1 -> Sum1/2
  Sum4/1 -> Sum1/1
  Math Function5/1 -> Sum4/1
  Product15/1 -> Sum4/2
  [A] -> Product15/2
  Sqrt2/1 -> Product15/1
  Constant14/1 -> Sqrt2/1
  [A] -> Math Function5/1
  Sum5/1 -> Product16/1
  Product7/1 -> Sum5/2
  Constant11/1 -> Product7/1
  Math Function4/1 -> Product7/2
  [A] -> Math Function4/1
  Constant6/1 -> Sum5/1
  Product11/1 -> b2/1, b0/1
  Constant10/1 -> Product11/1
  Constant2/1 -> Product1/1

== system tenneco_lib/ButterWorth Filters/Generic Low-Pass Filter/Stabilize Counter ==
  Compare To Constant1 : simulink/Logic and Bit Operations/Compare To Constant  relop=<  const=N  OutDataTypeStr=boolean
  Increment Counter : Subsystem
  Unit Delay2 : UnitDelay  InitialCondition=InitialCondition  SampleTime=-1  mask(Unit Delay){InitialCondition=0}
      mask prompts: InitialCondition "Simulink:blkprm_prompts:DelayBlkInitCond"
      mask help: Sample and hold with one sample period delay.
      mask TypeOptions InitialCondition: InitialCondition
  Stable : Outport  mask(Standard Outport){Port=1}
      mask prompts: Port "Simulink:blkprm_prompts:InOutportPortNum"
      mask help: Provide an output port for subsystems.
      mask TypeOptions Port: Port
  wires:
  Unit Delay2/1 -> Compare To Constant1/1, Increment Counter/1(x)
  Increment Counter/1(x+1) -> Unit Delay2/1
  Compare To Constant1/1 -> Stable/1, Increment Counter/Enable

== system tenneco_lib/ButterWorth Filters/Resettable Variable Low-Pass Filter/Stabilize Counter ==
  Compare To Constant1 : simulink/Logic and Bit Operations/Compare To Constant  relop=>=  const=N  OutDataTypeStr=boolean
  Increment Counter : Subsystem
  Logical Operator1 : Logic  Operator=NOT  Inputs=Inputs  AllPortsSameDT=off  OutDataTypeStr=boolean  mask(Logical Operator){Operator=NOT, Inputs=2}
      mask prompts: Operator "Simulink:blkprm_prompts:LogicOperator"; Inputs "Simulink:blkprm_prompts:LogicNumInputPorts"
      mask help: Logical operators. For a single input, operators are applied across the input vector. For multiple inputs, operators are applied across the inputs.
      mask TypeOptions Operator: Operator
      mask TypeOptions Inputs: Inputs
  Unit Delay : UnitDelay  InitialCondition=InitialCondition  SampleTime=-1  mask(Unit Delay){InitialCondition=0}
      mask prompts: InitialCondition "Simulink:blkprm_prompts:DelayBlkInitCond"
      mask help: Sample and hold with one sample period delay.
      mask TypeOptions InitialCondition: InitialCondition
  Stable : Outport  mask(Standard Outport){Port=1}
      mask prompts: Port "Simulink:blkprm_prompts:InOutportPortNum"
      mask help: Provide an output port for subsystems.
      mask TypeOptions Port: Port
  wires:
  Logical Operator1/1 -> Increment Counter/Enable
  Compare To Constant1/1 -> Logical Operator1/1, Stable/1
  Unit Delay/1 -> Compare To Constant1/1, Increment Counter/1(x)
  Increment Counter/1(x+1) -> Unit Delay/1

== system tenneco_lib/ButterWorth Filters/Variable Low-Pass Filter/Stabilize Counter ==
  Compare To Constant1 : simulink/Logic and Bit Operations/Compare To Constant  relop=>=  const=N  OutDataTypeStr=boolean
  Increment Counter : Subsystem
  Logical Operator1 : Logic  Operator=NOT  Inputs=Inputs  AllPortsSameDT=off  OutDataTypeStr=boolean  mask(Logical Operator){Operator=NOT, Inputs=2}
      mask prompts: Operator "Simulink:blkprm_prompts:LogicOperator"; Inputs "Simulink:blkprm_prompts:LogicNumInputPorts"
      mask help: Logical operators. For a single input, operators are applied across the input vector. For multiple inputs, operators are applied across the inputs.
      mask TypeOptions Operator: Operator
      mask TypeOptions Inputs: Inputs
  Unit Delay2 : UnitDelay  InitialCondition=InitialCondition  SampleTime=-1  mask(Unit Delay){InitialCondition=0}
      mask prompts: InitialCondition "Simulink:blkprm_prompts:DelayBlkInitCond"
      mask help: Sample and hold with one sample period delay.
      mask TypeOptions InitialCondition: InitialCondition
  Stable : Outport  mask(Standard Outport){Port=1}
      mask prompts: Port "Simulink:blkprm_prompts:InOutportPortNum"
      mask help: Provide an output port for subsystems.
      mask TypeOptions Port: Port
  wires:
  Increment Counter/1(x+1) -> Unit Delay2/1
  Unit Delay2/1 -> Compare To Constant1/1, Increment Counter/1(x)
  Compare To Constant1/1 -> Logical Operator1/1, Stable/1
  Logical Operator1/1 -> Increment Counter/Enable
